simulink model "SIM"  (R2022a)
settings: Solver=VariableStepAuto  StartTime=0.0  StopTime=Tsim  RelTol=1e-6  AbsTol=1e-9
values from neighbouring files (symbols this model uses):
  K = 0    [plotEnsayosPC.m]
  retraso = 0.06    [Fit_modelo.m]
libraries: cstblocks x1
settings Model: Creator=Francisco  LastModifiedBy=Francisco

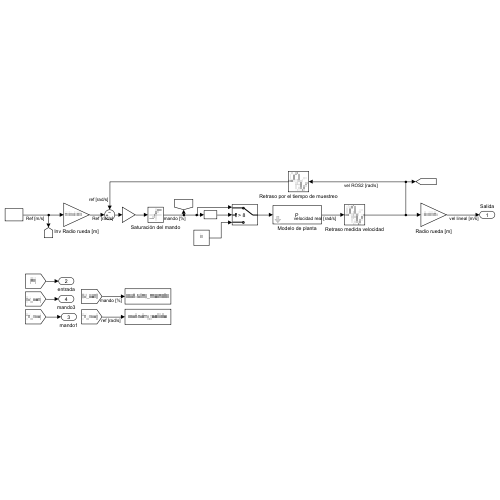
[thumbnail: Simulink's stored preview of the top-level diagram]
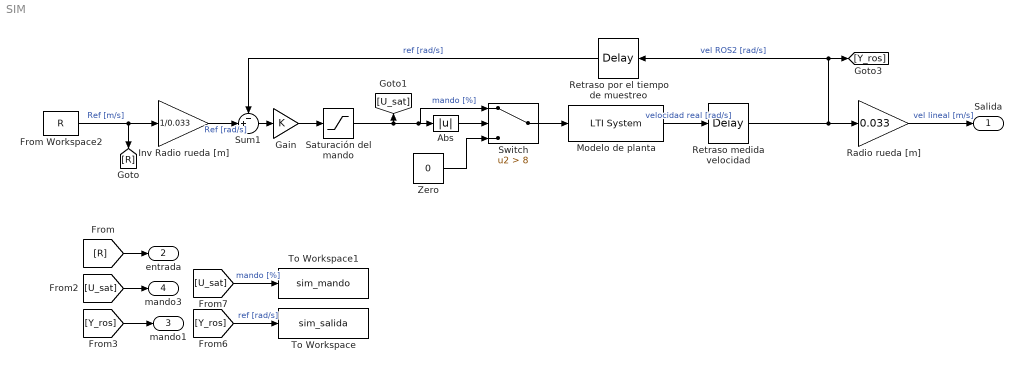
== system SIM ==
  Abs : Abs  SaturateOnIntegerOverflow=off
  From Workspace2 : FromWorkspace  VariableName=R  Interpolate=off  OutputAfterFinalValue=Holding final value
  Gain : Gain  Gain=K
  Inv Radio rueda [m] : Gain  Gain=1/0.033
  Modelo de planta : cstblocks/LTI System  sys=P  IC=[]
  Radio rueda [m] : Gain  Gain=0.033
  Retraso medida velocidad : TransportDelay  DelayTime=retraso  PadeOrder=2
  Retraso por el tiempo de muestreo : TransportDelay  DelayTime=0.015398/2
  Saturación del mando : Saturate  UpperLimit=100  LowerLimit=-100
  Sum1 : Sum  Inputs=-+|
  Switch : Switch  Criteria=u2 > Threshold  Threshold=8  SaturateOnIntegerOverflow=off  InputSameDT=off
  To Workspace : ToWorkspace  VariableName=sim_salida  SampleTime=-1
  To Workspace1 : ToWorkspace  VariableName=sim_mando  SampleTime=-1
  Zero : Constant  Value=0  OutDataTypeStr=Inherit: Inherit via back propagation
  Salida : Outport
  entrada : Outport  Port=2
  mando1 : Outport  Port=3
  mando3 : Outport  Port=4
  wires:
  Modelo de planta/1 -> Retraso medida velocidad/1  "velocidad real [rad/s]"
  Retraso por el tiempo de muestreo/1 -> Sum1/1  "ref [rad/s]"
  Saturación del mando/1 -> Abs/1, Switch/1, [U_sat]  "mando [%]"
  Retraso medida velocidad/1 -> Retraso por el tiempo de muestreo/1, [Y_ros], Radio rueda [m]/1  "vel ROS2 [rad/s]"
  Radio rueda [m]/1 -> Salida/1  "vel lineal [m/s]"
  Inv Radio rueda [m]/1 -> Sum1/2  "Ref [rad/s]"
  From Workspace2/1 -> Inv Radio rueda [m]/1, [R]  "Ref [m/s]"
  Sum1/1 -> Gain/1
  Gain/1 -> Saturación del mando/1
  [Y_ros] -> mando1/1
  [Y_ros] -> To Workspace/1  "ref [rad/s]"
  [U_sat] -> To Workspace1/1  "mando [%]"
  [R] -> entrada/1
  [U_sat] -> mando3/1
  Switch/1 -> Modelo de planta/1
  Abs/1 -> Switch/2
  Zero/1 -> Switch/3
